simulink model "BusCreatorBusSelector"  (Simulink 7.4)
settings: Solver=ode45  StartTime=0.0  StopTime=10.0  RelTol=1e-3
PostLoadFcn:
  | load Bus.mat
settings Model: Creator=dread  LastModifiedBy=dread

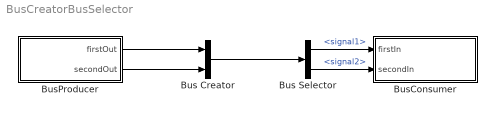
== system BusCreatorBusSelector ==
  Bus Creator : BusCreator  Inputs=2  UseBusObject=on
      settings: BusObject=Bus
  Bus Selector : BusSelector  OutputSignals=signal1,signal2
  BusConsumer : Subsystem
  BusProducer : Subsystem
  wires:
  BusProducer/1(firstOut) -> Bus Creator/1
  BusProducer/2(secondOut) -> Bus Creator/2
  Bus Selector/1 -> BusConsumer/1(firstIn)  "<signal1>"
  Bus Selector/2 -> BusConsumer/2(secondIn)  "<signal2>"
  Bus Creator/1 -> Bus Selector/1

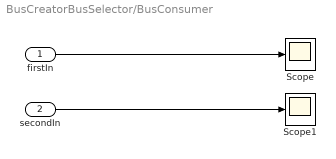
== system BusCreatorBusSelector/BusConsumer ==
  firstIn : Inport  OutDataType=fixdt(1, 16)  OutScaling=2^0
      settings: BusObject=Bus
  secondIn : Inport  Port=2  OutDataType=fixdt(1, 16)  OutScaling=2^0
  Scope : Scope
  Scope1 : Scope
  wires:
  firstIn/1 -> Scope/1
  secondIn/1 -> Scope1/1

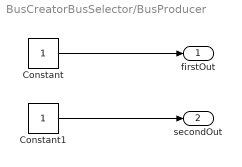
== system BusCreatorBusSelector/BusProducer ==
  Constant : Constant  OutDataType=fixdt(1, 16)  OutScaling=2^0
  Constant1 : Constant  OutDataType=fixdt(1, 16)  OutScaling=2^0
  firstOut : Outport  OutDataType=fixdt(1, 16)  OutScaling=2^0
  secondOut : Outport  Port=2  OutDataType=fixdt(1, 16)  OutScaling=2^0
  wires:
  Constant1/1 -> secondOut/1
  Constant/1 -> firstOut/1
